simulink model "SF033A_VehSigCdng"  (R2013b)
settings: Solver=FixedStepDiscrete  SolverMode=SingleTasking  StartTime=0.0  StopTime=1  FixedStep=.002  RelTol=1e-3
model workspace (MAT data in the model file):
  SLAMConfig_1_ATPP = [3707764736; 2; 1; 1; 1; 34]
values from neighbouring files (symbols this model uses):
  ARCHGLBPRM_2MILLISEC_SEC_F32 = DataDict.Constant    [SF033A_VehSigCdng_DataDict.m]
  ARCHGLBPRM_PIOVER180_ULS_F32 = DataDict.Constant    [SF033A_VehSigCdng_DataDict.m]
  AUNITCNVN_KPHPERSECPERMTRPERSECSQD_F32 = DataDict.Constant    [SF033A_VehSigCdng_DataDict.m]
  FLTINJ_VEHSIGCDNG_SERLCOMVEHLATA = DataDict.Constant    [SF033A_VehSigCdng_DataDict.m]
  FLTINJ_VEHSIGCDNG_SERLCOMVEHLGTA = DataDict.Constant    [SF033A_VehSigCdng_DataDict.m]
  FLTINJ_VEHSIGCDNG_SERLCOMVEHSPD = DataDict.Constant    [SF033A_VehSigCdng_DataDict.m]
  FLTINJ_VEHSIGCDNG_SERLCOMVEHYAWRATE = DataDict.Constant    [SF033A_VehSigCdng_DataDict.m]
  KPHCONVTOMTRPERSEC_MTRPERSECPERKPH_F32 = DataDict.Constant    [SF033A_VehSigCdng_DataDict.m]
  VehSigCdngDftLatA = DataDict.Calibration    [SF033A_VehSigCdng_DataDict.m]
  VehSigCdngDftLgtA = DataDict.Calibration    [SF033A_VehSigCdng_DataDict.m]
  VehSigCdngDftVehSpd = DataDict.Calibration    [SF033A_VehSigCdng_DataDict.m]
  VehSigCdngDftYawRate = DataDict.Calibration    [SF033A_VehSigCdng_DataDict.m]
  VehSigCdngLatADifThd = DataDict.Calibration    [SF033A_VehSigCdng_DataDict.m]
  VehSigCdngLatASlewRate = DataDict.Calibration    [SF033A_VehSigCdng_DataDict.m]
  VehSigCdngLtgADifThd = DataDict.Calibration    [SF033A_VehSigCdng_DataDict.m]
  VehSigCdngLtgASlewRate = DataDict.Calibration    [SF033A_VehSigCdng_DataDict.m]
  VehSigCdngVehSpdDifThd = DataDict.Calibration    [SF033A_VehSigCdng_DataDict.m]
  VehSigCdngVehSpdSlewRate = DataDict.Calibration    [SF033A_VehSigCdng_DataDict.m]
  VehSigCdngVehYawSlewRate = DataDict.Calibration    [SF033A_VehSigCdng_DataDict.m]
  VehSigCdngYawRateDifThd = DataDict.Calibration    [SF033A_VehSigCdng_DataDict.m]
  VEHSPDOVRDHWTQTHD_HWNWTMTR_F32 = DataDict.Constant    [SF033A_VehSigCdng_DataDict.m]
libraries: NxtrLim x9, CollectionOfReusableBlocks x6, Fil x4, simulink x1
(part 3 of 3)

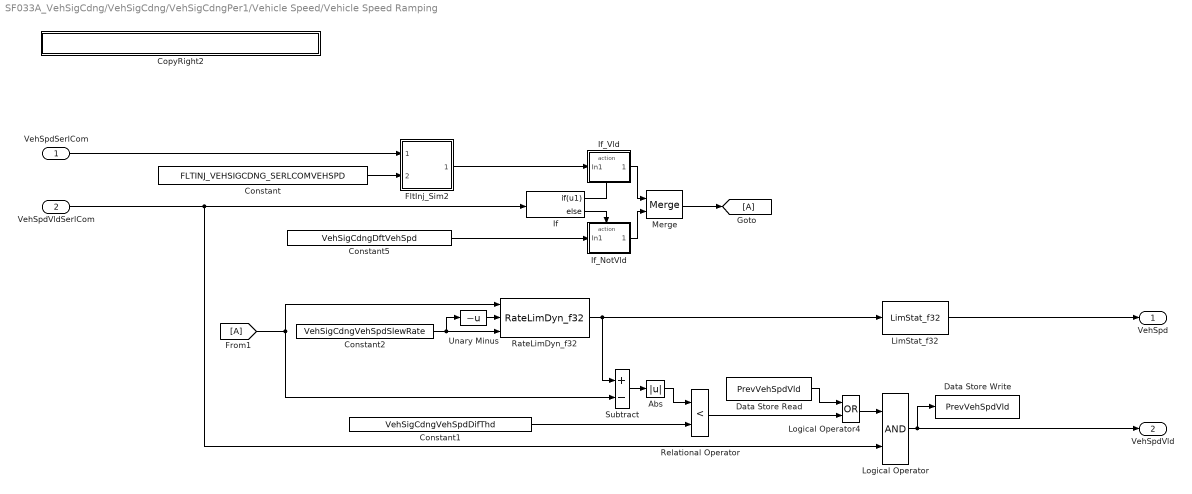
== system SF033A_VehSigCdng/VehSigCdng/VehSigCdngPer1/Vehicle Speed/Vehicle Speed Ramping ==
  VehSpdSerlCom : Inport  RequirementInfo="{'linktype_rmi_doors' '00012fc2 (/E-STEER Core/SubSystem Specifications/Application Functions - EA4/SF033A Vehicle Signal Conditioning)' '#SF033A_83' 'true' 'REQ:  SF033A_83' '' ; 'linktype_rmi_doors' '00012fc2 (/E-STEER Core/SubSystem Specifications/Application Functions - EA4/SF033A Vehicle Signal Conditioning)' '#SF033A_75' 'true' 'REQ:  SF033A_75' '' } %GIDa_a9d552c3_5684_4ee6_9dcd_40e111e11e6b"  PortDimensions=1
  VehSpdVldSerlCom : Inport  RequirementInfo="{'linktype_rmi_doors' '00012fc2 (/E-STEER Core/SubSystem Specifications/Application Functions - EA4/SF033A Vehicle Signal Conditioning)' '#SF033A_83' 'true' 'REQ:  SF033A_83' '' ; 'linktype_rmi_doors' '00012fc2 (/E-STEER Core/SubSystem Specifications/Application Functions - EA4/SF033A Vehicle Signal Conditioning)' '#SF033A_75' 'true' 'REQ:  SF033A_75' '' } %GIDa_ffec5aba_d673_4675_9949_6346e8150eda"  Port=2  PortDimensions=1
  Abs : Abs  RequirementInfo="{'linktype_rmi_doors' '00012fc2 (/E-STEER Core/SubSystem Specifications/Application Functions - EA4/SF033A Vehicle Signal Conditioning)' '#SF033A_77' 'true' 'REQ:  SF033A_77' '' } %GIDa_ff10e081_5597_4a74_80f9_545eb12ffbc4"
  Constant : Constant  RequirementInfo="{'linktype_rmi_doors' '00012fc2 (/E-STEER Core/SubSystem Specifications/Application Functions - EA4/SF033A Vehicle Signal Conditioning)' '#SF033A_107' 'true' 'REQ:  SF033A_107' '' } %GIDa_16fa97c2_e5e4_4133_946c_1f72cacbd852"  Value=FLTINJ_VEHSIGCDNG_SERLCOMVEHSPD
  Constant1 : Constant  RequirementInfo="{'linktype_rmi_doors' '00012fc2 (/E-STEER Core/SubSystem Specifications/Application Functions - EA4/SF033A Vehicle Signal Conditioning)' '#SF033A_77' 'true' 'REQ:  SF033A_77' '' } %GIDa_9e6fc4fd_eb84_4002_8a77_51454316c4ff"  Value=VehSigCdngVehSpdDifThd
  Constant2 : Constant  RequirementInfo="{'linktype_rmi_doors' '00012fc2 (/E-STEER Core/SubSystem Specifications/Application Functions - EA4/SF033A Vehicle Signal Conditioning)' '#SF033A_76' 'true' 'REQ:  SF033A_76' '' } %GIDa_153165e2_4d66_482c_bc70_f41e1bbccd2d"  Value=VehSigCdngVehSpdSlewRate
  Constant5 : Constant  RequirementInfo="{'linktype_rmi_doors' '00012fc2 (/E-STEER Core/SubSystem Specifications/Application Functions - EA4/SF033A Vehicle Signal Conditioning)' '#SF033A_75' 'true' 'REQ:  SF033A_75' '' } %GIDa_dadf8337_40e8_4abf_a657_3bf754b56750"  Value=VehSigCdngDftVehSpd
  CopyRight2 : Subsystem  Description=|  mask(Copyright Information){none=on}
      | Copyright info block.                                               
      |                                                                     
      | Place copyright information at the top of every subsystem in design.
      mask prompts: none "No parameters"
      mask help: Place copyright information at the top of every subsystem in design.
      mask Display:
      | NxtrConf = 'Nexteer Confidential';
      | 
      | sys = bdroot; %handle for the current model ("system")
      | first = get_param(sys,'Created');
      | first = first(end-3:end);  %year is last four digits
      | 
      | last = get_param(sys,'LastModifiedDate');
      | if isempty(last)
      |     last = datestr(now,'yyyy');
      | else
      |     last = last(end-3:end);
      | end
      | 
      | if strcmp(first,last)
      |     fprintf('%s -- Copyright %s Nexteer',NxtrConf,first)
      | else
      |     fprintf('%s -- %s%s- %s Nexteer',NxtrConf,char(169),first,last)
      | end
  Data Store Read : DataStoreRead  DataStoreName=PrevVehSpdVld
  Data Store Write : DataStoreWrite  DataStoreName=PrevVehSpdVld
  FltInj_Sim2 : Subsystem  RequirementInfo="{'linktype_rmi_doors' '00012fc2 (/E-STEER Core/SubSystem Specifications/Application Functions - EA4/SF033A Vehicle Signal Conditioning)' '#SF033A_107' 'true' 'REQ:  SF033A_107' '' } %GIDa_0a274aa2_d59c_4df8_99dd_f10073943b3d"  TreatAsAtomicUnit=on  VariantControl=FltInj_sim
  If : If  RequirementInfo="{'linktype_rmi_doors' '00012fc2 (/E-STEER Core/SubSystem Specifications/Application Functions - EA4/SF033A Vehicle Signal Conditioning)' '#SF033A_83' 'true' 'REQ:  SF033A_83' '' ; 'linktype_rmi_doors' '00012fc2 (/E-STEER Core/SubSystem Specifications/Application Functions - EA4/SF033A Vehicle Signal Conditioning)' '#SF033A_75' 'true' 'REQ:  SF033A_75' '' } %GIDa_262c624a_6210_497e_99a8_9380d2864317"  IfExpression=u1
  If_NotVld : Subsystem  RequirementInfo="{'linktype_rmi_doors' '00012fc2 (/E-STEER Core/SubSystem Specifications/Application Functions - EA4/SF033A Vehicle Signal Conditioning)' '#SF033A_75' 'true' 'REQ:  SF033A_75' '' } %GIDa_1d597542_a44a_4dad_9b6d_bd2c19164fdd"  TreatAsAtomicUnit=on
  If_Vld : Subsystem  RequirementInfo="{'linktype_rmi_doors' '00012fc2 (/E-STEER Core/SubSystem Specifications/Application Functions - EA4/SF033A Vehicle Signal Conditioning)' '#SF033A_83' 'true' 'REQ:  SF033A_83' '' } %GIDa_a9b0144d_d8f5_4d60_af55_f63e1b461c95"  TreatAsAtomicUnit=on
  LimStat_f32 : NxtrLim/LimStat_f32  RequirementInfo="{'linktype_rmi_doors' '00012fc2 (/E-STEER Core/SubSystem Specifications/Application Functions - EA4/SF033A Vehicle Signal Conditioning)' '#SF033A_68' 'true' 'REQ:  SF033A_68' '' } %GIDa_0f676263_5af2_454c_b342_7e84f6ef3f9d"  LoLim=VEHSPDMINLIM_KPH_F32  HiLim=VEHSPDMAXLIM_KPH_F32
      settings: AttributesFormatString=|
      | Low Limit: %<LoLim>
      | High Limit:%<HiLim>
  Logical Operator : Logic  RequirementInfo="{'linktype_rmi_doors' '00012fc2 (/E-STEER Core/SubSystem Specifications/Application Functions - EA4/SF033A Vehicle Signal Conditioning)' '#SF033A_77' 'true' 'REQ:  SF033A_77' '' } %GIDa_98d87574_5a46_468e_8909_cbe598971a8f"  AllPortsSameDT=off  OutDataTypeStr=boolean
  Logical Operator4 : Logic  RequirementInfo={} %GIDa_2e0a24a1_ca47_474d_9722_1a543d763886  Operator=OR  AllPortsSameDT=off  OutDataTypeStr=boolean
  Merge : Merge  RequirementInfo="{'linktype_rmi_doors' '00012fc2 (/E-STEER Core/SubSystem Specifications/Application Functions - EA4/SF033A Vehicle Signal Conditioning)' '#SF033A_75' 'true' 'REQ:  SF033A_75' '' ; 'linktype_rmi_doors' '00012fc2 (/E-STEER Core/SubSystem Specifications/Application Functions - EA4/SF033A Vehicle Signal Conditioning)' '#SF033A_83' 'true' 'REQ:  SF033A_83' '' } %GIDa_5a04fb05_6550_474d_bf4b_85be5d4efad6"
  RateLimDyn_f32 : NxtrLim/RateLimDyn_f32  RequirementInfo="{'linktype_rmi_doors' '00012fc2 (/E-STEER Core/SubSystem Specifications/Application Functions - EA4/SF033A Vehicle Signal Conditioning)' '#SF033A_76' 'true' 'REQ:  SF033A_76' '' ; 'linktype_rmi_doors' '00012fc2 (/E-STEER Core/SubSystem Specifications/Application Functions - EA4/SF033A Vehicle Signal Conditioning)' '#SF033A_77' 'true' 'REQ:  SF033A_77' '' } %GIDa_a35ef298_c6c0_4dc7_a84e_48fb3049ae58"  StVar=PrevVehSpd  Ts=ARCHGLBPRM_2MILLISEC_SEC_F32
      settings: AttributesFormatString=StVar: %<StVar>
  Relational Operator : RelationalOperator  RequirementInfo="{'linktype_rmi_doors' '00012fc2 (/E-STEER Core/SubSystem Specifications/Application Functions - EA4/SF033A Vehicle Signal Conditioning)' '#SF033A_77' 'true' 'REQ:  SF033A_77' '' } %GIDa_f4c6bc09_2cce_4926_820b_b2f188311d69"  Operator=<  OutDataTypeStr=boolean
  Subtract : Sum  RequirementInfo="{'linktype_rmi_doors' '00012fc2 (/E-STEER Core/SubSystem Specifications/Application Functions - EA4/SF033A Vehicle Signal Conditioning)' '#SF033A_77' 'true' 'REQ:  SF033A_77' '' } %GIDa_b0052b3d_e826_4390_8299_ea5316a8a12b"  Inputs=+-
  Unary Minus : UnaryMinus  RequirementInfo="{'linktype_rmi_doors' '00012fc2 (/E-STEER Core/SubSystem Specifications/Application Functions - EA4/SF033A Vehicle Signal Conditioning)' '#SF033A_76' 'true' 'REQ:  SF033A_76' '' } %GIDa_b8db9cbd_94bf_4430_ac3d_004558f5147d"
  VehSpd : Outport  RequirementInfo="{'linktype_rmi_doors' '00012fc2 (/E-STEER Core/SubSystem Specifications/Application Functions - EA4/SF033A Vehicle Signal Conditioning)' '#SF033A_83' 'true' 'REQ:  SF033A_83' '' ; 'linktype_rmi_doors' '00012fc2 (/E-STEER Core/SubSystem Specifications/Application Functions - EA4/SF033A Vehicle Signal Conditioning)' '#SF033A_75' 'true' 'REQ:  SF033A_75' '' } %GIDa_0d7361b7_fecf_473d_881b_29d3abeb8efe"
  VehSpdVld : Outport  RequirementInfo="{'linktype_rmi_doors' '00012fc2 (/E-STEER Core/SubSystem Specifications/Application Functions - EA4/SF033A Vehicle Signal Conditioning)' '#SF033A_83' 'true' 'REQ:  SF033A_83' '' ; 'linktype_rmi_doors' '00012fc2 (/E-STEER Core/SubSystem Specifications/Application Functions - EA4/SF033A Vehicle Signal Conditioning)' '#SF033A_75' 'true' 'REQ:  SF033A_75' '' } %GIDa_15c422ee_8510_4435_9ce8_8fae2591f2b1"  Port=2
  wires:
  Subtract/1 -> Abs/1
  Abs/1 -> Relational Operator/1
  Constant1/1 -> Relational Operator/2
  Constant/1 -> FltInj_Sim2/2(Enum)
  LimStat_f32/1 -> VehSpd/1
  [A] -> Subtract/2, RateLimDyn_f32/1
  Logical Operator4/1 -> Logical Operator/1
  Relational Operator/1 -> Logical Operator4/2
  Data Store Read/1 -> Logical Operator4/1
  If/1 -> If_Vld/Action
  If/2 -> If_NotVld/Action
  If_Vld/1(Out1) -> Merge/1
  If_NotVld/1(Out1) -> Merge/2
  Merge/1 -> [A]
  VehSpdVldSerlCom/1 -> Logical Operator/2, If/1
  FltInj_Sim2/1(Out1) -> If_Vld/1(In1)
  Constant5/1 -> If_NotVld/1(In1)
  Constant2/1 -> Unary Minus/1, RateLimDyn_f32/3
  Unary Minus/1 -> RateLimDyn_f32/2
  RateLimDyn_f32/1 -> LimStat_f32/1, Subtract/1
  Logical Operator/1 -> Data Store Write/1, VehSpdVld/1
  VehSpdSerlCom/1 -> FltInj_Sim2/1(Signal)

== system SF033A_VehSigCdng/VehSigCdng/VehSigCdngPer1/Yaw Rate /CopyRight2 ==

== system SF033A_VehSigCdng/VehSigCdng/VehSigCdngPer1/Yaw Rate /FltInj_Sim ==
  note: This block requires no modification by FDD author.
      |
      | This block does not actually simulate any fault injection.  It is simply a pass-thru.
      |
      | The Enum port (#2) simply terminates its signal, but we are trying to force the FDD author
      | to properly use the FltInjectionLocType enumeration in FDD model.
  note: EA4.x Fault Injection
  note: Inport #2 must be enumeration
      | Enum: FltInjectionLocType
  Signal : Inport
  Enum : Inport  Port=2
  CopyRight2 : CollectionOfReusableBlocks/CopyRight2  Description=|  none=on
      | Copyright info block.                                               
      |                                                                     
      | Place copyright information at the top of every subsystem in design.
  Terminator : Terminator
  Out1 : Outport
  wires:
  Signal/1 -> Out1/1
  Enum/1 -> Terminator/1

== system SF033A_VehSigCdng/VehSigCdng/VehSigCdngPer1/Yaw Rate /If_NotVld ==
  In1 : Inport
  Action Port : ActionPort  ActionType=else
  CopyRight2 : Subsystem  Description=|  mask(Copyright Information){none=on}
      | Copyright info block.                                               
      |                                                                     
      | Place copyright information at the top of every subsystem in design.
      mask prompts: none "No parameters"
      mask help: Place copyright information at the top of every subsystem in design.
      mask Display:
      | NxtrConf = 'Nexteer Confidential';
      | 
      | sys = bdroot; %handle for the current model ("system")
      | first = get_param(sys,'Created');
      | first = first(end-3:end);  %year is last four digits
      | 
      | last = get_param(sys,'LastModifiedDate');
      | if isempty(last)
      |     last = datestr(now,'yyyy');
      | else
      |     last = last(end-3:end);
      | end
      | 
      | if strcmp(first,last)
      |     fprintf('%s -- Copyright %s Nexteer',NxtrConf,first)
      | else
      |     fprintf('%s -- %s%s- %s Nexteer',NxtrConf,char(169),first,last)
      | end
  Out1 : Outport
  wires:
  In1/1 -> Out1/1

== system SF033A_VehSigCdng/VehSigCdng/VehSigCdngPer1/Yaw Rate /If_Vld ==
  In1 : Inport
  Action Port : ActionPort  ActionType=then
  CopyRight2 : Subsystem  Description=|  mask(Copyright Information){none=on}
      | Copyright info block.                                               
      |                                                                     
      | Place copyright information at the top of every subsystem in design.
      mask prompts: none "No parameters"
      mask help: Place copyright information at the top of every subsystem in design.
      mask Display:
      | NxtrConf = 'Nexteer Confidential';
      | 
      | sys = bdroot; %handle for the current model ("system")
      | first = get_param(sys,'Created');
      | first = first(end-3:end);  %year is last four digits
      | 
      | last = get_param(sys,'LastModifiedDate');
      | if isempty(last)
      |     last = datestr(now,'yyyy');
      | else
      |     last = last(end-3:end);
      | end
      | 
      | if strcmp(first,last)
      |     fprintf('%s -- Copyright %s Nexteer',NxtrConf,first)
      | else
      |     fprintf('%s -- %s%s- %s Nexteer',NxtrConf,char(169),first,last)
      | end
  Out1 : Outport
  wires:
  In1/1 -> Out1/1

== system SF033A_VehSigCdng/VehSigCdng/VehSigCdngPer1/Lateral Acceleration/If_Vld/CopyRight2 ==

== system SF033A_VehSigCdng/VehSigCdng/VehSigCdngPer1/Lateral Acceleration/if_NotVld/CopyRight2 ==

== system SF033A_VehSigCdng/VehSigCdng/VehSigCdngPer1/Longitudinal Acceleration/If_NotVld/CopyRight2 ==

== system SF033A_VehSigCdng/VehSigCdng/VehSigCdngPer1/Longitudinal Acceleration/If_Vld/CopyRight2 ==

== system SF033A_VehSigCdng/VehSigCdng/VehSigCdngPer1/Vehicle Speed/No_VehSpd_Override/CopyRight2 ==

== system SF033A_VehSigCdng/VehSigCdng/VehSigCdngPer1/Vehicle Speed/VehSpd_Override/CopyRight2 ==

== system SF033A_VehSigCdng/VehSigCdng/VehSigCdngPer1/Vehicle Speed/Vehicle Speed Ramping/CopyRight2 ==

== system SF033A_VehSigCdng/VehSigCdng/VehSigCdngPer1/Vehicle Speed/Vehicle Speed Ramping/FltInj_Sim2 ==
  note: This block requires no modification by FDD author.
      |
      | This block does not actually simulate any fault injection.  It is simply a pass-thru.
      |
      | The Enum port (#2) simply terminates its signal, but we are trying to force the FDD author
      | to properly use the FltInjectionLocType enumeration in FDD model.
  note: EA4.x Fault Injection
  note: Inport #2 must be enumeration
      | Enum: FltInjectionLocType
  Signal : Inport
  Enum : Inport  Port=2
  CopyRight2 : CollectionOfReusableBlocks/CopyRight2  Description=|  none=on
      | Copyright info block.                                               
      |                                                                     
      | Place copyright information at the top of every subsystem in design.
  Terminator : Terminator
  Out1 : Outport
  wires:
  Signal/1 -> Out1/1
  Enum/1 -> Terminator/1

== system SF033A_VehSigCdng/VehSigCdng/VehSigCdngPer1/Vehicle Speed/Vehicle Speed Ramping/If_NotVld ==
  In1 : Inport
  Action Port : ActionPort  ActionType=else
  CopyRight2 : Subsystem  Description=|  mask(Copyright Information){none=on}
      | Copyright info block.                                               
      |                                                                     
      | Place copyright information at the top of every subsystem in design.
      mask prompts: none "No parameters"
      mask help: Place copyright information at the top of every subsystem in design.
      mask Display:
      | NxtrConf = 'Nexteer Confidential';
      | 
      | sys = bdroot; %handle for the current model ("system")
      | first = get_param(sys,'Created');
      | first = first(end-3:end);  %year is last four digits
      | 
      | last = get_param(sys,'LastModifiedDate');
      | if isempty(last)
      |     last = datestr(now,'yyyy');
      | else
      |     last = last(end-3:end);
      | end
      | 
      | if strcmp(first,last)
      |     fprintf('%s -- Copyright %s Nexteer',NxtrConf,first)
      | else
      |     fprintf('%s -- %s%s- %s Nexteer',NxtrConf,char(169),first,last)
      | end
  Out1 : Outport
  wires:
  In1/1 -> Out1/1

== system SF033A_VehSigCdng/VehSigCdng/VehSigCdngPer1/Vehicle Speed/Vehicle Speed Ramping/If_Vld ==
  In1 : Inport
  Action Port : ActionPort  ActionType=then
  CopyRight2 : Subsystem  Description=|  mask(Copyright Information){none=on}
      | Copyright info block.                                               
      |                                                                     
      | Place copyright information at the top of every subsystem in design.
      mask prompts: none "No parameters"
      mask help: Place copyright information at the top of every subsystem in design.
      mask Display:
      | NxtrConf = 'Nexteer Confidential';
      | 
      | sys = bdroot; %handle for the current model ("system")
      | first = get_param(sys,'Created');
      | first = first(end-3:end);  %year is last four digits
      | 
      | last = get_param(sys,'LastModifiedDate');
      | if isempty(last)
      |     last = datestr(now,'yyyy');
      | else
      |     last = last(end-3:end);
      | end
      | 
      | if strcmp(first,last)
      |     fprintf('%s -- Copyright %s Nexteer',NxtrConf,first)
      | else
      |     fprintf('%s -- %s%s- %s Nexteer',NxtrConf,char(169),first,last)
      | end
  Out1 : Outport
  wires:
  In1/1 -> Out1/1

== system SF033A_VehSigCdng/VehSigCdng/VehSigCdngPer1/Yaw Rate /If_NotVld/CopyRight2 ==

== system SF033A_VehSigCdng/VehSigCdng/VehSigCdngPer1/Yaw Rate /If_Vld/CopyRight2 ==

== system SF033A_VehSigCdng/VehSigCdng/VehSigCdngPer1/Vehicle Speed/Vehicle Speed Ramping/If_NotVld/CopyRight2 ==

== system SF033A_VehSigCdng/VehSigCdng/VehSigCdngPer1/Vehicle Speed/Vehicle Speed Ramping/If_Vld/CopyRight2 ==
